simulink model "H_neuralnet_incomplete"  (R2017a)
settings: Solver=VariableStepAuto  StartTime=0.0  StopTime=200  FixedStep=0.01  RelTol=1e-3  EnableMultiTasking=on
libraries: dspsrcs4 x4
settings Model: Creator=markvoskuijl  LastModifiedBy=Luca
settings DataIOCC: LimitDataPoints=on  SaveFormat=Array  SignalLoggingSaveFormat=ModelDataLogs
settings OptimizationCC: ExpressionDepthLimit=2147483647  LifeSpan=inf
settings DebuggingCC: UnderspecifiedInitializationDetection=Classic  MergeDetectMultiDrivingBlocksExec=none  SolverPrmCheckMsg=warning  FcnCallInpInsideContextMsg=warning  StateNameClashWarn=warning  SFUnexpectedBacktrackingDiag=warning  SFNoUnconditionalDefaultTransitionDiag=warning  SFExecutionAtInitializationDiag=none
settings HardwareCC: ProdBitPerPointer=32  ProdBitPerSizeT=32  ProdBitPerPtrDiffT=32  ProdLargestAtomicFloat=None  ProdIntDivRoundTo=Undefined  ProdEndianess=Unspecified  ProdWordSize=32  ProdHWDeviceType=32-bit Generic
settings ModelReferenceCC: PropagateSignalLabelsOutOfModel=off
settings GRTTargetCC: TargetLangStandard=C89/C90 (ANSI)  GeneratePreprocessorConditionals=Disable all  CombineOutputUpdateFcns=off  GRTInterface=on
settings ConfigComp: CovMetricSettings=dw  CovHtmlReporting=on  CovSaveCumulativeToWorkspaceVar=on  CovSaveSingleToWorkspaceVar=on  CovExternalEMLEnable=off

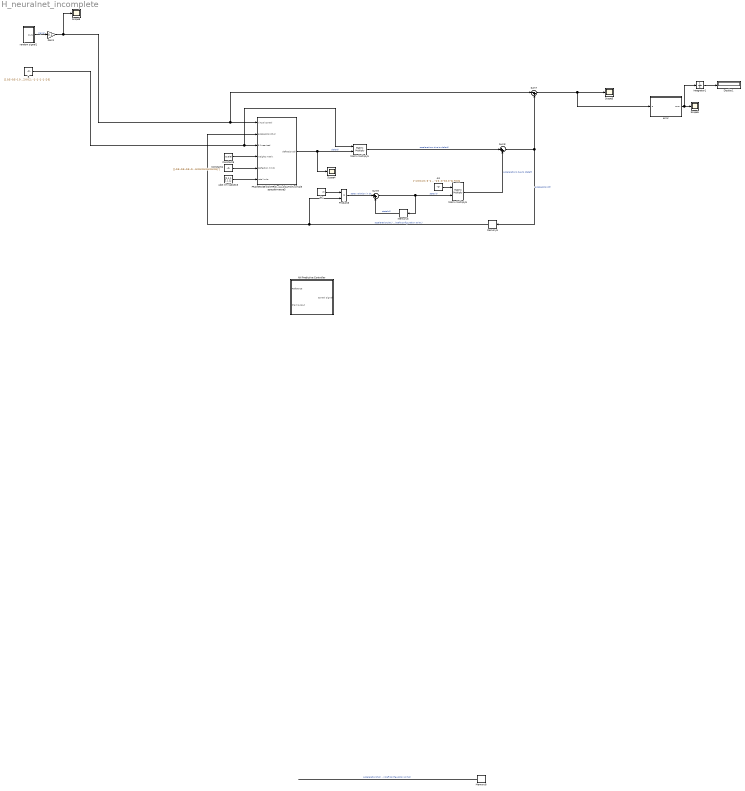
== system H_neuralnet_incomplete ==
  A3 : Constant  Value=[-1 0 0.1 0 ; 0 -1 0 -0.1 ; 0 0 -1 0 ; 0 -0.1 0 -1] *0.01
  B : Constant  Value=[1 0.5 -0.5 -1 0 0.05 ; 0 0 0 0 2 0 ; -0.02 -0.01 0.01 0.02 0 0.2 ; -1 -1 -1 -1 -2 0]
  Constant4 : Constant  Value=[[-0.5 -0.5 -0.5 -0.5 -0.5 -0.5].' [0.5 0.5 0.5 0.5 0.5 0.5].']
  Constant6 : Constant  Value=eye(6)
  Display1 : Display
  FRAMEWISE CONTROL ALLOCATION simple pseudoinverse3 : Subsystem
  Gain1 : Gain  Gain=0.1
  Integrator1 : Integrator
  Matrix Multiply5 : Product  Multiplication=Matrix(*)
  Matrix Multiply6 : Product  Multiplication=Matrix(*)
  Memory3 : Memory  X0=[0 0 0 0]
  Memory6 : Memory  X0=[0 0 0 0]
  Memory8 : Memory  X0=[0 0 0 0]
  NN Predictive Controller : Subsystem  mask(NN Predictive Controller){N2=7, Nu=2, Ts=0.2, rho=0.05, alpha=0.001, csrchfun=csrchbac, maxiter=2, S1=7, Ni=2, Nj=2, sim_file=cstr, trainfun=trainlm, Use_validation=1, Use_Testing=0, max_i=4, min_i=0, sam_training=8000, epochs=200, minp=0.02233575679015197, maxp=3.977181962055679, mint=19.990542740630676, maxt=23.003707300214998, Normalize=0, IW=[-20.531997924598212 18.706482494882994;0.0041681487931733516 -0.003898180117493663;0.0027271331329927679 -0.0026383962298670975;-4.2884263047654887 -2.5242458681173563;-7.5376751481296909 11.798966620249038;0.12631450792955951 0.63090781487873226;-9.0327138502332947 3.9557193990027328], LW1_2=[14.94314250694182 -17.959099344431603;-0.81834808440118445 0.41655850750692763;0.364433114947604 -0.17752308649608817;55.505918973874849 -51.271996485446365;-3.4857289415608221 2.5155674023943493;-1.0383681172774319 -0.1649807357299794;-1.7354318305331962 4.1593615744767991], LW2_1=[0.0026508898559841616 -1.0458797145936556 5.0292698388067745 0.00010141072535827776 0.0032962551987542432 0.58061299674354561 8.9082702971420182e-005], B1=[18.565258582766731;9.6542761594756836;-3.6577882481482806;-67.658021555936102;-2.7052627837062393;0.46399572090641622;-40.321245764315009], B2=21.149686119715415, max_i_int=20, min_i_int=5, limit_output=1, max_output=23, min_output=20, Use_Previous_Weights=1}
      mask prompts: Ts "Sample time"; rho "rho (typically = 0.03)"; alpha "alpha (typically = 0.001)"; csrchfun "Minimization rutine"; trainfun "Training function"
      mask help: NN Predictive Controller. You first train a neural network model of the plant to be controlled. The controller uses the plant model to predict plant performance over a specified time horizon. An optimization algorithm determines the control signal that optimizes plant performance over this horizon. Double click the NN Predictive Controller block to train the plant model and set the controller parameters.
      mask init:
      | xl = [0   .53   .53     .85   .85  .53  .53  NaN .85  .92 .92];
      | yl = [.95 .95 1.05  1.05   .82  .82  .95  NaN  .95 .95 .65];
      | x2 = [0 .53    NaN .92 1.2 NaN .53 .85 .85 .53 .53 ];
      | y2 = [.39 .39   NaN .65 .65 NaN .59 .59 .29 .29  .59];
      | x3 = [.67 .67 NaN .64 .67 .70 NaN .53 .4   .4   .53 NaN .46 .53 .46];
      | y3 = [.59 .82 NaN .66 .59 .66 NaN .55 .55 .86 .86 NaN  .89 .86 .83];
      | 
      | x1t=.03; y1t=.31;
      | x2t=.03; y2t=.8;
      | x8t=.03;y8t=.21;
      | x3t=.77; y3t=.53;
      | x4t=.77; y4t=.44;
      | x5t=.45; y5t=.76;
      | x6t=.45; y6t=.35;
      | x7t=.45; y7t=.25;
      settings: OpenFcn=nncontrolutil('nnpredict','',gcbh,gcb);
      mask TypeOptions csrchfun: csrchgol | csrchbac | csrchhyb | csrchbre | csrchcha
      mask TypeOptions trainfun: trainbfg | trainbr  | traincgb | traincgf | traincgp | traingd | traingdm | traingda | traingdx | trainlm  | trainoss | trainrp  | trainscg
      mask Display:
      | plot([[xl NaN x2]*.9-.075 ], [[yl  NaN y2]*.9-.1 ]);
      | plot([[x3]*.9-.075 ], [[y3]*.9-.1 ]);
      | text(x1t,y1t,'Plant');
      | text(x8t,y8t,'Output');
      | text(x2t,y2t,'Reference');
      | text(x3t,y3t,'Control');
      | text(x4t,y4t,'Signal');
      | text(x5t,y5t,'Optim.');
      | text(x6t,y6t,'NN');
      | text(x7t,y7t,'Model');
  Product3 : Product
  Scope{3..5,8} (4 alike) : Scope
  Sum7 : Sum  Inputs=|-+
  Sum8 : Sum  Inputs=|++
  Sum9 : Sum  Inputs=|++
  dt2 : Subsystem
  error : MATLAB Function  TreatAsAtomicUnit=on
  random signal1 : Subsystem
  udot lim rad/sec3 : Constant  Value=[1 1 1 1 1 1]
  wires:
  random signal1/1(Out1) -> Gain1/1  "signal"
  dt2/1(dt) -> Product3/1
  Sum8/1 -> Memory6/1, Sum7/2  "accelerations(t)"
  FRAMEWISE CONTROL ALLOCATION simple pseudoinverse3/1(deflections(t)) -> Scope4/1, Matrix Multiply5/2  "delta(t)"
  Matrix Multiply6/1 -> Sum8/2  "accelerations due to state(t)"
  udot lim rad/sec3/1 -> FRAMEWISE CONTROL ALLOCATION simple pseudoinverse3/6(rate limits)
  A3/1 -> Matrix Multiply6/1
  Memory6/1 -> FRAMEWISE CONTROL ALLOCATION simple pseudoinverse3/2(accelerations(t-1)), Product3/2  "accelerations(t-1) due to aircraft configuration at (t-1)"
  Memory3/1 -> Sum9/2  "state(t-1)"
  Constant4/1 -> FRAMEWISE CONTROL ALLOCATION simple pseudoinverse3/5(deflection limits)
  Product3/1 -> Sum9/1  "state variation in dt"
  Sum9/1 -> Matrix Multiply6/2, Memory3/1  "state (t)"
  Matrix Multiply5/1 -> Sum8/1  "accelerations due to delta(t)"
  Constant6/1 -> FRAMEWISE CONTROL ALLOCATION simple pseudoinverse3/4(weights matrix)
  error/1(error) -> Integrator1/1, Scope5/1
  Sum7/1 -> error/1(e), Scope3/1
  Integrator1/1 -> Display1/1
  Gain1/1 -> Sum7/1, FRAMEWISE CONTROL ALLOCATION simple pseudoinverse3/1(virtual control), Scope8/1
  B/1 -> Matrix Multiply5/1, FRAMEWISE CONTROL ALLOCATION simple pseudoinverse3/3(B linearized)
  Memory8/1 -> ?  "accelerations(t-1) due to aircraft configuration at (t-1)"

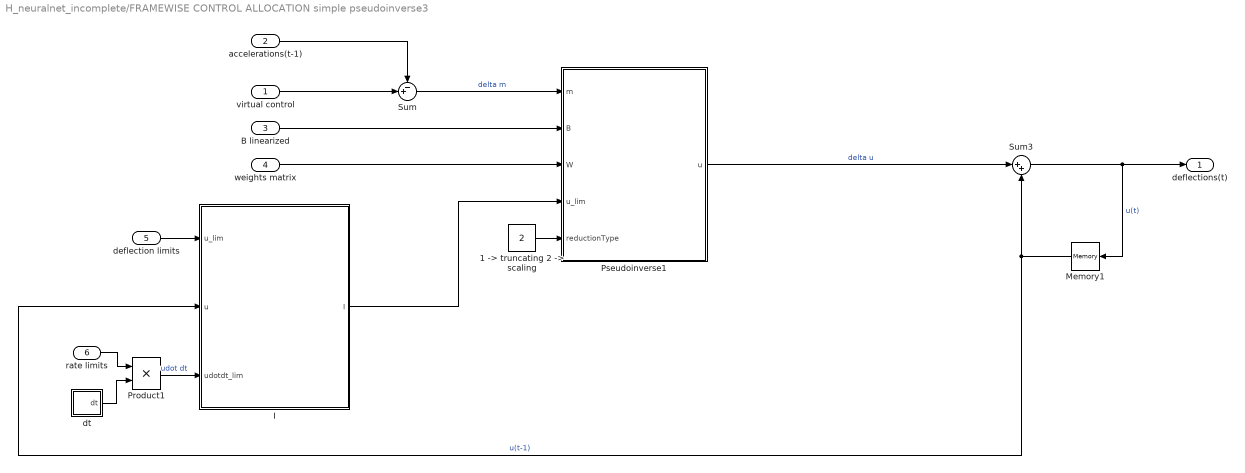
== system H_neuralnet_incomplete/FRAMEWISE CONTROL ALLOCATION simple pseudoinverse3 ==
  virtual control : Inport
  accelerations(t-1) : Inport  Port=2
  B linearized : Inport  Port=3
  weights matrix : Inport  Port=4
  deflection limits : Inport  Port=5
  rate limits : Inport  Port=6
  "1 -> truncating 2 -> scaling" : Constant  Value=2
  I : MATLAB Function  TreatAsAtomicUnit=on
  Memory1 : Memory
  Product1 : Product
  Pseudoinverse1 : MATLAB Function  TreatAsAtomicUnit=on
  Sum : Sum  Inputs=-+|
  Sum3 : Sum  Inputs=|++
  dt : Subsystem
  deflections(t) : Outport
  wires:
  I/1(I) -> Pseudoinverse1/4(u_lim)
  Memory1/1 -> I/2(u), Sum3/2  "u(t-1)"
  Product1/1 -> I/3(udotdt_lim)  "udot dt"
  rate limits/1 -> Product1/1
  Sum3/1 -> deflections(t)/1, Memory1/1  "u(t)"
  Pseudoinverse1/1(u) -> Sum3/1  "delta u"
  dt/1(dt) -> Product1/2
  B linearized/1 -> Pseudoinverse1/2(B)
  deflection limits/1 -> I/1(u_lim)
  weights matrix/1 -> Pseudoinverse1/3(W)
  "1 -> truncating 2 -> scaling"/1 -> Pseudoinverse1/5(reductionType)
  accelerations(t-1)/1 -> Sum/1
  virtual control/1 -> Sum/2
  Sum/1 -> Pseudoinverse1/1(m)  "delta m"

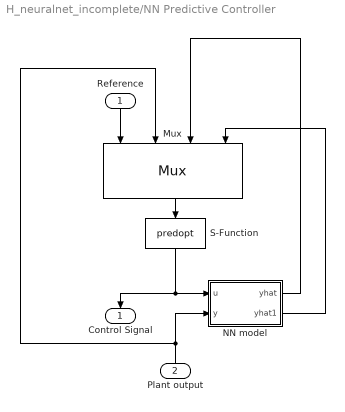
== system H_neuralnet_incomplete/NN Predictive Controller ==
  Reference : Inport
  Plant output : Inport  Port=2
  Mux : Mux
      settings: DisplayOption=signals
  NN model : Subsystem
  S-Function : S-Function  FunctionName=predopt  Parameters=N2,Ts,Nu,maxiter,csrchfun,rho,alpha,S1,IW,LW1_2,LW2_1,B1,B2,Ni,Nj,min_i,max_i,minp,maxp,mint,maxt,Normalize  SFunctionDeploymentMode=off  EnableBusSupport=off
  Control Signal : Outport
  wires:
  Mux/1 -> S-Function/1
  S-Function/1 -> NN model/1(u), Control Signal/1
  NN model/2(yhat1) -> Mux/4
  NN model/1(yhat) -> Mux/3
  Reference/1 -> Mux/1
  Plant output/1 -> NN model/2(y), Mux/2

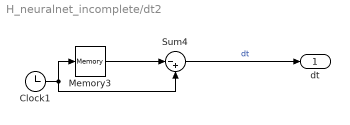
== system H_neuralnet_incomplete/dt2 ==
  Clock1 : Clock
  Memory3 : Memory
  Sum4 : Sum  Inputs=|-+
  dt : Outport
  wires:
  Clock1/1 -> Sum4/2, Memory3/1
  Memory3/1 -> Sum4/1
  Sum4/1 -> dt/1  "dt"

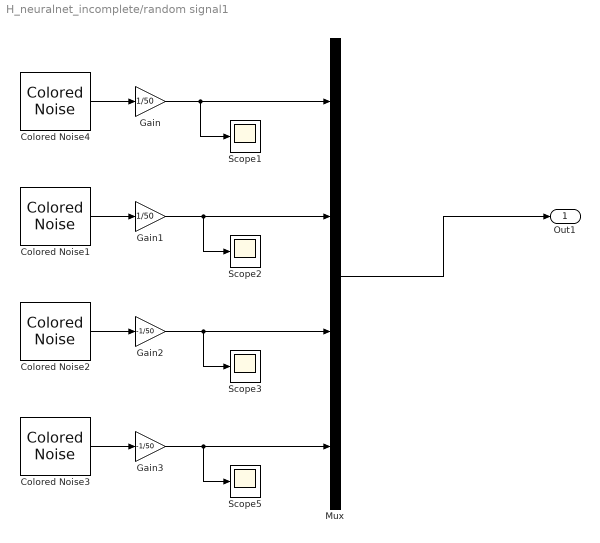
== system H_neuralnet_incomplete/random signal1 ==
  Colored Noise1 : dspsrcs4/Colored Noise  Color=custom  InverseFrequencyPower=2  NumChannels=1  OutputDataType=single  SamplesPerFrame=1  SampleTime=0.1  RandomStream=mt19937ar with seed  Seed=74  SimulateUsing=Interpreted execution
      settings: SourceProductName=DSP System Toolbox  SourceProductBaseCode=DS
  Colored Noise2 : dspsrcs4/Colored Noise  Color=custom  InverseFrequencyPower=2  NumChannels=1  OutputDataType=single  SamplesPerFrame=1  SampleTime=0.1  RandomStream=mt19937ar with seed  Seed=7  SimulateUsing=Interpreted execution
      settings: SourceProductName=DSP System Toolbox  SourceProductBaseCode=DS
  Colored Noise3 : dspsrcs4/Colored Noise  Color=custom  InverseFrequencyPower=2  NumChannels=1  OutputDataType=single  SamplesPerFrame=1  SampleTime=0.1  RandomStream=mt19937ar with seed  Seed=55  SimulateUsing=Interpreted execution
      settings: SourceProductName=DSP System Toolbox  SourceProductBaseCode=DS
  Colored Noise4 : dspsrcs4/Colored Noise  Color=custom  InverseFrequencyPower=2  NumChannels=1  OutputDataType=single  SamplesPerFrame=1  SampleTime=0.1  RandomStream=mt19937ar with seed  Seed=56  SimulateUsing=Interpreted execution
      settings: SourceProductName=DSP System Toolbox  SourceProductBaseCode=DS
  Gain : Gain  Gain=1/50
  Gain1 : Gain  Gain=1/50
  Gain2 : Gain  Gain=-1/50
  Gain3 : Gain  Gain=-1/50
  Mux : Mux
  Scope{1..3,5} (4 alike) : Scope
  Out1 : Outport
  wires:
  Colored Noise4/1 -> Gain/1
  Colored Noise1/1 -> Gain1/1
  Colored Noise2/1 -> Gain2/1
  Gain/1 -> Scope1/1, Mux/1
  Gain1/1 -> Scope2/1, Mux/2
  Gain2/1 -> Scope3/1, Mux/3
  Mux/1 -> Out1/1
  Gain3/1 -> Mux/4, Scope5/1
  Colored Noise3/1 -> Gain3/1

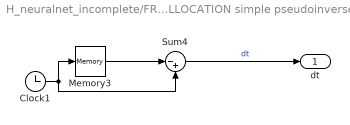
== system H_neuralnet_incomplete/FRAMEWISE CONTROL ALLOCATION simple pseudoinverse3/dt ==
  Clock1 : Clock
  Memory3 : Memory
  Sum4 : Sum  Inputs=|-+
  dt : Outport
  wires:
  Clock1/1 -> Sum4/2, Memory3/1
  Memory3/1 -> Sum4/1
  Sum4/1 -> dt/1  "dt"

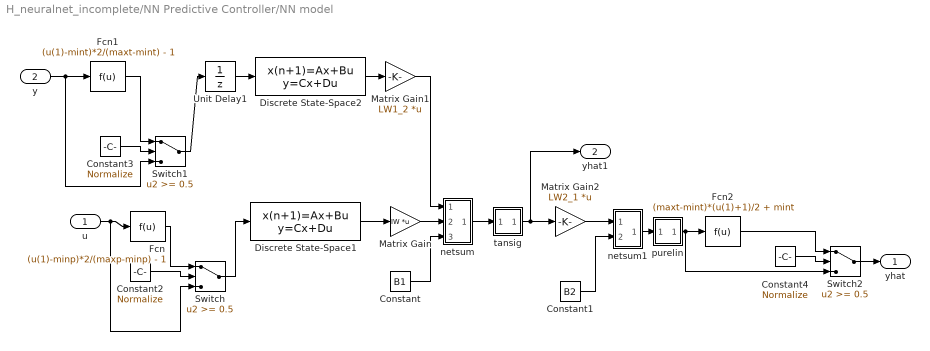
== system H_neuralnet_incomplete/NN Predictive Controller/NN model ==
  u : Inport
  y : Inport  Port=2
  Constant : Constant  Value=B1
  Constant1 : Constant  Value=B2
  Constant2 : Constant  Value=Normalize
  Constant3 : Constant  Value=Normalize
  Constant4 : Constant  Value=Normalize
  Discrete State-Space1 : DiscreteStateSpace  A=[0 zeros(1,Ni-2);eye(Ni-2,Ni-1)]  B=[zeros(double(Ni==1));eye(Ni-1,1)]  C=[0 zeros(1,Ni-2);eye(Ni-1,Ni-1)]  D=eye(Ni,1)  SampleTime=Ts
  Discrete State-Space2 : DiscreteStateSpace  A=[0 zeros(1,Nj-2);eye(Nj-2,Nj-1)]  B=[zeros(double(Nj==1));eye(Nj-1,1)]  C=[0 zeros(1,Nj-2);eye(Nj-1,Nj-1)]  D=eye(Nj,1)  SampleTime=Ts
  Fcn : Fcn  Expr=(u(1)-minp)*2/(maxp-minp) - 1
  Fcn1 : Fcn  Expr=(u(1)-mint)*2/(maxt-mint) - 1
  Fcn2 : Fcn  Expr=(maxt-mint)*(u(1)+1)/2 + mint
  Matrix Gain : Gain  Gain=IW  Multiplication=Matrix(K*u)  SaturateOnIntegerOverflow=on  OutDataTypeStr=Inherit: Same as input  ParamDataTypeStr=Inherit: Same as input
  Matrix Gain1 : Gain  Gain=LW1_2  Multiplication=Matrix(K*u)  SaturateOnIntegerOverflow=on  OutDataTypeStr=Inherit: Same as input  ParamDataTypeStr=Inherit: Same as input
  Matrix Gain2 : Gain  Gain=LW2_1  Multiplication=Matrix(K*u)  SaturateOnIntegerOverflow=on  OutDataTypeStr=Inherit: Same as input  ParamDataTypeStr=Inherit: Same as input
  Switch : Switch  Threshold=0.5  ZeroCross=off  SaturateOnIntegerOverflow=on  InputSameDT=on
  Switch1 : Switch  Threshold=0.5  ZeroCross=off  SaturateOnIntegerOverflow=on  InputSameDT=on
  Switch2 : Switch  Threshold=0.5  ZeroCross=off  SaturateOnIntegerOverflow=on  InputSameDT=on
  Unit Delay1 : UnitDelay  SampleTime=Ts
  netsum : Subsystem
      mask Display: disp('+')
  netsum1 : Subsystem
      mask Display: disp('+')
  purelin : Subsystem
      mask Display: plot([-1 1],[0 0],[-1 1],[-1 1])
  tansig : Subsystem
      mask Display: plot([-1 1],[0 0],[-1 -.9 -.8 -.7 -.6 -.5 -.4 -.3 -.2 -.1 0 .1 .2 .3 .4 .5 .6 .7 .8 .9 1],2./(1+exp(-8*[-1 -.9 -.8 -.7 -.6 -.5 -.4 -.3 -.2 -.1 0 .1 .2 .3 .4 .5 .6 .7 .8 .9 1]))-1)
  yhat : Outport
  yhat1 : Outport  Port=2
  wires:
  netsum1/1(Out1) -> purelin/1(n)
  Constant1/1 -> netsum1/2(In2)
  Matrix Gain2/1 -> netsum1/1(In1)
  netsum/1(Out1) -> tansig/1(n)
  Constant/1 -> netsum/3(In3)
  Matrix Gain1/1 -> netsum/1(In1)
  Matrix Gain/1 -> netsum/2(In2)
  tansig/1(a) -> Matrix Gain2/1, yhat1/1
  Discrete State-Space1/1 -> Matrix Gain/1
  Fcn/1 -> Switch/1
  Switch/1 -> Discrete State-Space1/1
  u/1 -> Fcn/1, Switch/3
  Constant2/1 -> Switch/2
  Discrete State-Space2/1 -> Matrix Gain1/1
  Unit Delay1/1 -> Discrete State-Space2/1
  Constant3/1 -> Switch1/2
  Switch1/1 -> Unit Delay1/1
  Fcn1/1 -> Switch1/1
  y/1 -> Fcn1/1, Switch1/3
  Constant4/1 -> Switch2/2
  Switch2/1 -> yhat/1
  Fcn2/1 -> Switch2/1
  purelin/1(a) -> Fcn2/1, Switch2/3

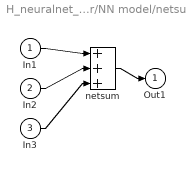
== system H_neuralnet_incomplete/NN Predictive Controller/NN model/netsum ==
  In1 : Inport
  In2 : Inport  Port=2
  In3 : Inport  Port=3
  netsum : Sum  Inputs=3  SaturateOnIntegerOverflow=on  InputSameDT=on  OutDataTypeStr=Inherit: Same as first input
  Out1 : Outport
  wires:
  In1/1 -> netsum/1
  In2/1 -> netsum/2
  In3/1 -> netsum/3
  netsum/1 -> Out1/1

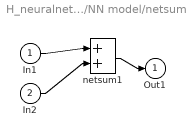
== system H_neuralnet_incomplete/NN Predictive Controller/NN model/netsum1 ==
  In1 : Inport
  In2 : Inport  Port=2
  netsum1 : Sum  Inputs=2  SaturateOnIntegerOverflow=on  InputSameDT=on  OutDataTypeStr=Inherit: Same as first input
  Out1 : Outport
  wires:
  In1/1 -> netsum1/1
  In2/1 -> netsum1/2
  netsum1/1 -> Out1/1

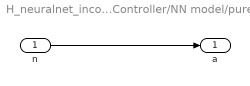
== system H_neuralnet_incomplete/NN Predictive Controller/NN model/purelin ==
  n : Inport
  a : Outport
  wires:
  n/1 -> a/1

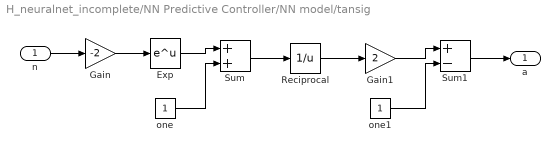
== system H_neuralnet_incomplete/NN Predictive Controller/NN model/tansig ==
  n : Inport
  Exp : Math  SaturateOnIntegerOverflow=on
  Gain : Gain  Gain=-2  SaturateOnIntegerOverflow=on  OutDataTypeStr=Inherit: Same as input  ParamDataTypeStr=Inherit: Same as input
  Gain1 : Gain  Gain=2  SaturateOnIntegerOverflow=on  OutDataTypeStr=Inherit: Same as input  ParamDataTypeStr=Inherit: Same as input
  Reciprocal : Math  Operator=reciprocal  SaturateOnIntegerOverflow=on
  Sum : Sum  SaturateOnIntegerOverflow=on  InputSameDT=on  OutDataTypeStr=Inherit: Same as first input
  Sum1 : Sum  Inputs=+-  SaturateOnIntegerOverflow=on  InputSameDT=on  OutDataTypeStr=Inherit: Same as first input
  one : Constant
  one1 : Constant
  a : Outport
  wires:
  n/1 -> Gain/1
  Gain/1 -> Exp/1
  Exp/1 -> Sum/1
  one/1 -> Sum/2
  Sum/1 -> Reciprocal/1
  Reciprocal/1 -> Gain1/1
  Gain1/1 -> Sum1/1
  one1/1 -> Sum1/2
  Sum1/1 -> a/1

== matlab function H_neuralnet_incomplete/FRAMEWISE CONTROL ALLOCATION simple pseudoinverse3/I ==
  data: u_lim input; u input; udotdt_lim input; I output
function I = computeIntersection(u_lim, u, udotdt_lim)
%check if the matrices are correct
    if not(isequal(size(u_lim,1),size(udotdt_lim,1), size(u,1)))
        error ('input matrix dimensions do not match')
    end

%declare space of intersection
    I = zeros(length(u_lim),2);
    
    I(:,1) = -min(udotdt_lim, abs(u_lim(:,1)-u));
    I(:,2) = min(+udotdt_lim, u_lim(:,2)-u);
    
end

== matlab function H_neuralnet_incomplete/FRAMEWISE CONTROL ALLOCATION simple pseudoinverse3/Pseudoinverse1 ==
  data: m input; u output; B input; W input; u_lim input; reductionType input
function u = Pseudoinverse(m, B, W, u_lim, reductionType)
coder.varsize('u_index', 'Br', 'Wr', 'u_sat');

%check if the matrices are correct
    if not(isequal(size(u_lim,1),size(B,2),size(W,1),size(W,2))...
       && isequal(length(m),size(B,1)))
        error ('input matrix dimensions do not match')
    end
    
%assign to every equation an index    
    u_index = [1:length(u_lim)].';
    
%check the type of system and then compute the pseudoinverse 1st step
    order = size(B,2)-size(B,1);

    if order > 0 %over-determined, solution that minimizes the 2norm
        u = inv(W)*B'*inv(B*inv(W)*B')*m;
    elseif order < 0 %under-determined, solution that minimizes the error
        u = inv(B'*B)*B'*m;   
    else %order = 0, sqared thus invertiBrle
        u = inv(B)*m;
    end

%deifne u_sat vector
    u_sat = zeros(length(u),1);
    
%check if the first iteration solution is correct then return    
    if not(any(u < u_lim(:,1))||any(u > u_lim(:,2)))  
        return
    end
    
%The software continues only if the solution has to be reduced
%reduce their value
    switch reductionType
        case 1 %truncation
            %takes note of which one are out of their bounds
                u_sat(u < u_lim(:,1)) = 1;
                u_sat(u > u_lim(:,2)) = 1;
                
            %trucate
                u = min(u, u_lim(:,2));
                u = max(u, u_lim(:,1));

        case 2 %scaling solution -> direction preserving
            %reduce
                a = zeros(length(u),1);

                for i = 1:length(u)
                    if u(i)>0
                       a(i) = abs(u(i)/u_lim(i,2));
                    elseif u(i)<0
                       a(i) = abs(u(i)/u_lim(i,1));
                    else
                       a(i) = 0; 
                    end          
                end
                a_max = max(a);
                u = u/a_max;
            
            %takes note of which one are out of their bounds
                u_sat(u == u_lim(:,2)) = 1;
                u_sat(u == u_lim(:,1)) = 1;
            
    end
    
return
    
end

== matlab function H_neuralnet_incomplete/error ==
  data: e input; error output
function error = error(e)

    error = sum(abs(e));

end
